simulink model "blockdemo"  (Simulink 6.3)
settings: Solver=ode45  StartTime=0.0  StopTime=20  RelTol=1e-3
InitFcn:
  | %% DSPBuilder Start
  | alt_dspbuilder_update_model(bdroot)
  | %% DSPBuilder End
libraries: allblocks_alteradspbuilder2 x6
settings Model: Creator=cpurcell  LastModifiedBy=delphick
settings DebuggingCC: MultiTaskDSMMsg=error

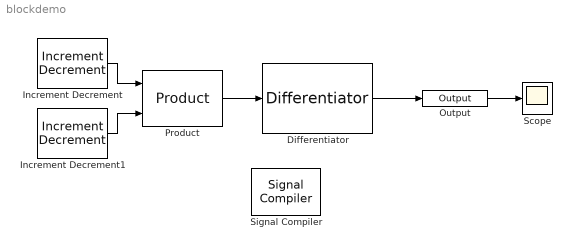
== system blockdemo ==
  Differentiator : allblocks_alteradspbuilder2/Differentiator  bwl=16  depth=1  use_ena=off  use_sclr=off
  Increment Decrement : allblocks_alteradspbuilder2/Increment Decrement  BusType=Signed Integer  bwl=8  bwr=8  SpecifyClock=off  clr_value=0  direction=Increment  phase_selection=1  use_ena=off  use_sclr=off
  Increment Decrement1 : allblocks_alteradspbuilder2/Increment Decrement  BusType=Signed Integer  bwl=8  bwr=8  SpecifyClock=off  clr_value=0  direction=Increment  phase_selection=1  use_ena=off  use_sclr=off
  Output : allblocks_alteradspbuilder2/Output  iofile=C:\workspace_clean\Documentation\DesignExamples\Tutorials\UnitBlocks\Arithmetic\Differentiator\tb_blockdemo\blockdemo_Output.capture  BusType=Signed Integer  bwl=8  bwr=0  PORTTYPE=Output
  Product : allblocks_alteradspbuilder2/Product  BusType=Inferred  bwl=8  bwr=0  pipeline=0  phase_selection=1  use_ena=off  use_aclr=off  UseLPM=off  UseDedicatedCircuitry=off
  Scope : Scope
      settings: TimeRange=20  YMin=-1  YMax=40
  Signal Compiler : allblocks_alteradspbuilder2/Signal Compiler  DeviceFamily=Stratix IV  DeviceName=AUTO  EnableSignalTap=off  SignalTapDepth=128  UseBoardBlock=off  StpUseDefaultClock=on  StpClock=clock
  wires:
  Increment Decrement/1 -> Product/1
  Increment Decrement1/1 -> Product/2
  Product/1 -> Differentiator/1
  Differentiator/1 -> Output/1
  Output/1 -> Scope/1
